simulink model "RT_ctrl_analyse1"  (R2013a)
settings: Solver=ode45  StartTime=0.0  StopTime=10.0  RelTol=1e-3
settings Model: Creator=mainster  LastModifiedBy=mainster
settings DebuggingCC: SolverPrmCheckMsg=none

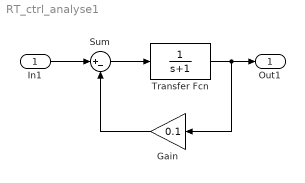
== system RT_ctrl_analyse1 ==
  In1 : Inport
  Gain : Gain  Gain=0.1
  Sum : Sum  Inputs=|+-
  Transfer Fcn : TransferFcn  Denominator=[1 1]
  Out1 : Outport
  wires:
  In1/1 -> Sum/1
  Sum/1 -> Transfer Fcn/1
  Gain/1 -> Sum/2
  Transfer Fcn/1 -> Gain/1, Out1/1
